simulink model "untitled"  (R2025a)
settings: Solver=VariableStepAuto  StartTime=0.0  StopTime=10.0  RelTol=1e-3
settings Model: Creator=nikul  LastModifiedBy=nikul

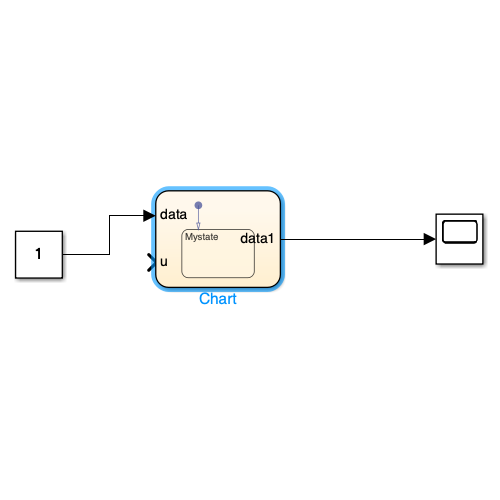
[thumbnail: Simulink's stored preview of the top-level diagram]
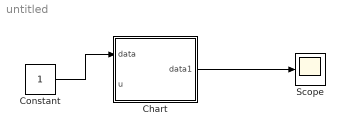
== system untitled ==
  Chart : Stateflow chart  TreatAsAtomicUnit=on
  Constant : Constant
  Scope : Scope
  wires:
  Constant/1 -> Chart/1(data)
  Chart/1(data1) -> Scope/1

== stateflow chart untitled/Chart ==
  state Mystate
  (default) -> Mystate
  data: data input; data1 output; u input
